simulink model "R_SIPsim"  (R2021b)
settings: Solver=ode45  StartTime=0.0  StopTime=10.0  FixedStep=0.01  RelTol=1e-3
settings Model: Creator=Utente  LastModifiedBy=Utente

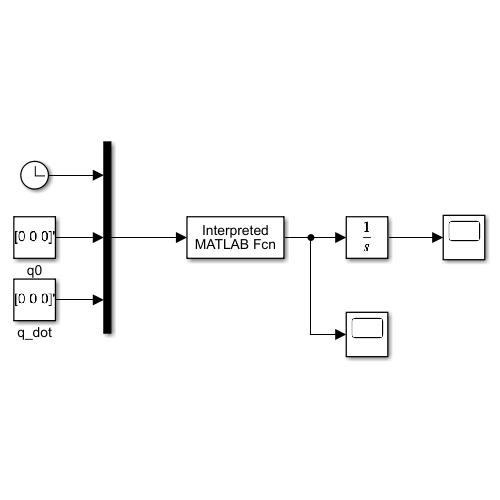
[thumbnail: Simulink's stored preview of the top-level diagram]
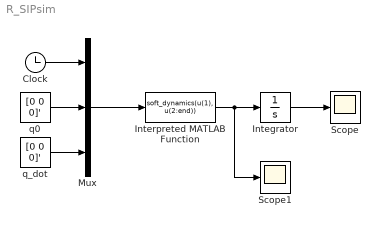
== system R_SIPsim ==
  Clock : Clock
  Integrator : Integrator  InitialCondition=zeros(6, 1)
  Interpreted MATLAB Function : MATLABFcn  MATLABFcn=soft_dynamics(u(1), u(2:end))
  Mux : Mux  Inputs=3
  Scope : Scope
  Scope1 : Scope
  q0 : Constant  Value=[0 0 0]'
  q_dot : Constant  Value=[0 0 0]'
  wires:
  q0/1 -> Mux/2
  q_dot/1 -> Mux/3
  Mux/1 -> Interpreted MATLAB Function/1
  Clock/1 -> Mux/1
  Interpreted MATLAB Function/1 -> Scope1/1, Integrator/1
  Integrator/1 -> Scope/1
